simulink model "DC_Motor"  (R2018b)
settings: Solver=VariableStepAuto  StartTime=0.0  StopTime=10  RelTol=1e-3
values from neighbouring files (symbols this model uses):
  b = 22.5    [DC_Simulink.m]
  J = 2.21E-6    (= 2.21e-06)    [DC_Servomotor_Code.m]    (also in DC_Simulink.m = 0.306)
  K = 0.055    [DC_Servomotor_Code.m]    (also in DC_Simulink.m = 0.109)
  L = 5.02E-3    (= 0.00502)    [DC_Servomotor_Code.m]    (also in DC_Simulink.m = 0.000625)
  R = 41.5    [DC_Servomotor_Code.m]    (also in DC_Simulink.m = 0.522)
  Tload = TL(1,i)    [DC_Simulink.m]
libraries: simulink x1
settings Model: Creator=James  LastModifiedBy=James

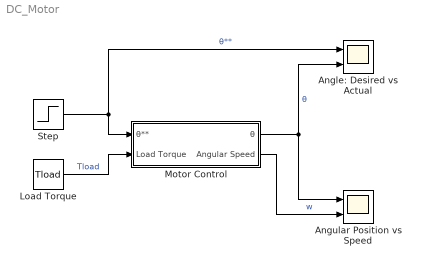
== system DC_Motor ==
  Angle: Desired vs Actual : Scope  NumInputPorts=2
  Angular Position vs Speed : Scope  NumInputPorts=2
  Load Torque : Constant  Value=Tload
  Motor Control : Subsystem
  Step : Step  SampleTime=0
  wires:
  Step/1 -> Motor Control/1(θ**), Angle: Desired vs Actual/1  "θ**"
  Motor Control/1(θ) -> Angle: Desired vs Actual/2, Angular Position vs Speed/1  "θ"
  Motor Control/2(Angular Speed) -> Angular Position vs Speed/2  "w"
  Load Torque/1 -> Motor Control/2(Load Torque)  "Tload"

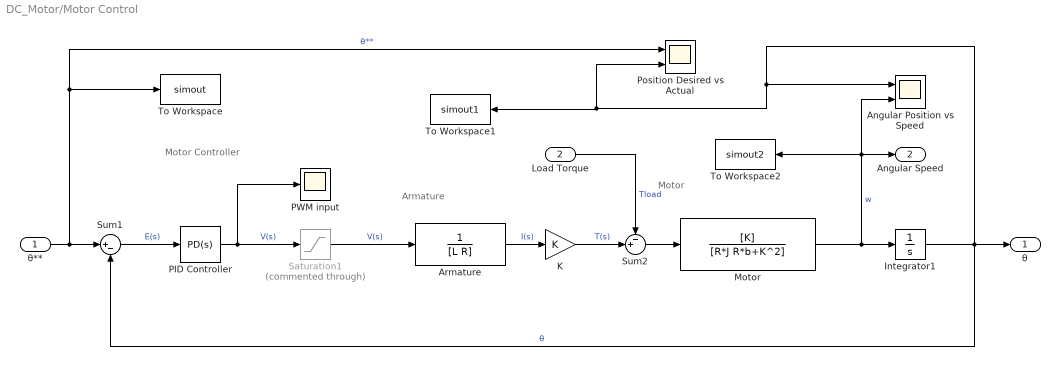
== system DC_Motor/Motor Control ==
  note: Armature
  note: Motor
  note: Motor Controller
  θ** : Inport
  Load Torque : Inport  Port=2
  Angular Position vs Speed : Scope  NumInputPorts=2
  Armature : TransferFcn  Denominator=[L R]
  Integrator1 : Integrator
  K : Gain  Gain=K
  Motor : TransferFcn  Numerator=[K]  Denominator=[R*J R*b+K^2]
  PID Controller : simulink/Continuous/PID Controller  Controller=PD  Form=Parallel  TimeDomain=Continuous-time  SampleTime=-1  IntegratorMethod=Forward Euler  FilterMethod=Forward Euler  ControllerParametersSource=internal  P=360670.773162426  I=648207.462988784  D=5632.57342733881  UseFilter=on  N=72854.7210023152  TunerSelectOption=Transfer Function Based (PID Tuner App)  InitialConditionSource=internal  InitialConditionForIntegrator=0  InitialConditionForFilter=0  DifferentiatorICPrevScaledInput=0  ExternalReset=none  TrackingMode=off  Kt=1  LimitOutput=off  UpperSaturationLimit=inf  LowerSaturationLimit=-inf  LinearizeAsGain=on  AntiWindupMode=none  Kb=1  POutMin=[]  POutMax=[]  IOutMin=[]  IOutMax=[]  DOutMin=[]  DOutMax=[]  NOutMin=[]  NOutMax=[]  SumOutMin=[]  SumOutMax=[]  SaturationOutMin=[]  SaturationOutMax=[]  PParamMin=[]  PParamMax=[]  IParamMin=[]  IParamMax=[]  DParamMin=[]  DParamMax=[]  NParamMin=[]  NParamMax=[]  KbParamMin=[]  KbParamMax=[]  KtParamMin=[]  KtParamMax=[]  KbOutMin=[]  KbOutMax=[]  KtOutMin=[]  KtOutMax=[]  IntegratorOutMin=[]  IntegratorOutMax=[]  FilterOutMin=[]  FilterOutMax=[]  SumI1OutMin=[]  SumI1OutMax=[]  SumI2OutMin=[]  SumI2OutMax=[]  SumI3OutMin=[]  SumI3OutMax=[]  SumI4OutMin=[]  SumI4OutMax=[]  SumDOutMin=[]  SumDOutMax=[]  DifferentiatorOutMin=[]  DifferentiatorOutMax=[]  FilterDiffOutCoefMin=[]  FilterDiffOutCoefMax=[]  ReciprocalOutMin=[]  ReciprocalOutMax=[]  SumDenOutMin=[]  SumDenOutMax=[]  SumNumOutMin=[]  SumNumOutMax=[]  DivideOutMin=[]  DivideOutMax=[]  IntegratorContinuousStateAttributes=''  IntegratorStateMustResolveToSignalObject=off  IntegratorRTWStateStorageClass=Auto  FilterContinuousStateAttributes=''  FilterStateMustResolveToSignalObject=off  FilterRTWStateStorageClass=Auto  ParallelPVariant=InternalParameters  IdealPVariant=Disabled  IVariant=Disabled  DVariant=InternalParameters  IntegratorVariant=Disabled  SatVariant=Disabled  AWVariant=Disabled  PCopyVariant=Disabled  TRVariant=Disabled  FdbkBlocksVariant=Forward  IdealPFdbkVariant=Disabled  SatFdbkVariant=Disabled  DerivativeFilterVariant=ContFilter  NVariant=InternalParameters  NCopyVariant=Disabled  FilterICVariant=InternalICsFilter  IntegratorICVariant=Disabled  ExternalResetVariant=Disabled  TRSumVariant=Passthrough  SumFdbkVariant=Disabled  SumVariant=Sum_PD
  PWM input : Scope
  Position Desired vs Actual : Scope  NumInputPorts=2
  Saturation1 : Saturate  Commented=through  UpperLimit=127  LowerLimit=-127
  Sum1 : Sum  Inputs=|+-
  Sum2 : Sum  Inputs=-+|
  To Workspace : ToWorkspace  VariableName=simout  SaveFormat=Timeseries  SampleTime=-1
  To Workspace1 : ToWorkspace  VariableName=simout1  SaveFormat=Timeseries  SampleTime=-1
  To Workspace2 : ToWorkspace  VariableName=simout2  SaveFormat=Timeseries  SampleTime=-1
  θ : Outport
  Angular Speed : Outport  Port=2
  wires:
  Sum2/1 -> Motor/1
  Motor/1 -> Integrator1/1, Angular Position vs Speed/2, To Workspace2/1, Angular Speed/1  "w"
  Integrator1/1 -> θ/1, Sum1/2, To Workspace1/1, Position Desired vs Actual/2, Angular Position vs Speed/1  "θ"
  Load Torque/1 -> Sum2/1  "Tload"
  Sum1/1 -> PID Controller/1  "E(s)"
  PID Controller/1 -> PWM input/1, Saturation1/1  "V(s)"
  K/1 -> Sum2/2  "T(s)"
  Armature/1 -> K/1  "I(s)"
  θ**/1 -> To Workspace/1, Position Desired vs Actual/1, Sum1/1  "θ**"
  Saturation1/1 -> Armature/1  "V(s)"
